simulink model "Tim1PWM_Tim3IC"  (R2018b)
settings: Solver=FixedStepDiscrete  StartTime=0.0  StopTime=10.0  FixedStep=0.5  RelTol=1e-3  EnableMultiTasking=on
libraries: USART_Lib x4, TIMERS_Lib x2, STM32_Config_Lib x1
settings Model: Creator=Gang  LastModifiedBy=fenard1
settings DataIOCC: LimitDataPoints=on  SaveFormat=Array
settings OptimizationCC: DefaultParameterBehavior=Inlined  DefaultUnderspecifiedDataType=single  PassReuseOutputArgsAs=Individual arguments  LifeSpan=1
settings DebuggingCC: UnderspecifiedInitializationDetection=Classic  MergeDetectMultiDrivingBlocksExec=none  SolverPrmCheckMsg=warning  UniqueDataStoreMsg=error  AssertControl=DisableAll  AllowSymbolicDim=off  StrictBusMsg=ErrorOnBusTreatedAsVector  SFUnexpectedBacktrackingDiag=warning  SFNoUnconditionalDefaultTransitionDiag=warning  SFUndirectedBroadcastEventsDiag=error  SFExecutionAtInitializationDiag=none
settings HardwareCC: ProdBitPerPointer=32  ProdBitPerSizeT=32  ProdBitPerPtrDiffT=32  ProdLargestAtomicInteger=Integer  ProdWordSize=32  ProdHWDeviceType=STMicroelectronics->STM32 32-bit Cortex-M
settings ModelReferenceCC: PropagateSignalLabelsOutOfModel=off
settings SFSimCC: SimUseLocalCustomCode=off  CompileTimeRecursionLimit=0  EnableRuntimeRecursion=off  MATLABDynamicMemAlloc=off
settings RTWCC: SystemTargetFile=stm32.tlc  TemplateMakefile=stm32.tmf  Description=stm32 (Embedded Target)  GenerateReport=on  RTWUseLocalCustomCode=off
settings CodeAppCC: IgnoreCustomStorageClasses=off  CustomSymbolStrType=$N$R$M  SimulinkBlockComments=off
settings STFCustomTargetCC: TargetLangStandard=C99 (ISO)  ParMdlRefBuildCompliant=on  IncludeMdlTerminateFcn=off  CombineOutputUpdateFcns=on  ERTCustomFileBanners=on  SupportComplex=off  SupportContinuousTime=off  SupportNonInlinedSFcns=off  RemoveResetFunc=on  ParenthesesLevel=Maximum  CastingMode=Standards  MATLABClassNameForMDSCustomization=Simulink.SoftwareTarget.ERTCustomization  SystemTargetFile=stm32.tlc
settings ERTTargetCC: TargetLangStandard=C99 (ISO)  MultiwordLength=2048  CompOptLevelCompliant=off  ConcurrentExecutionCompliant=off  IncludeMdlTerminateFcn=off  SupportComplex=off  ParenthesesLevel=Maximum  CastingMode=Standards  ModelStepFunctionPrototypeControlCompliant=off  CPPClassGenCompliant=off  UseToolchainInfoCompliant=off  ERTSrcFileBannerTemplate=sourceFileTemplate.cgt  ERTHdrFileBannerTemplate=sourceFileTemplate.cgt  ERTDataSrcFileTemplate=sourceFileTemplate.cgt  ERTDataHdrFileTemplate=sourceFileTemplate.cgt  ERTCustomFileTemplate=customRoutineProcess.tlc  ConvertIfToSwitch=off  SuppressUnreachableDefaultCases=off  EnableSignedLeftShifts=off  EnableSignedRightShifts=off
settings ConfigComp: CovMetricSettings=dw  CovHtmlReporting=on  CovSaveCumulativeToWorkspaceVar=on  CovSaveSingleToWorkspaceVar=on  CovExternalEMLEnable=off  CovSFcnEnable=off

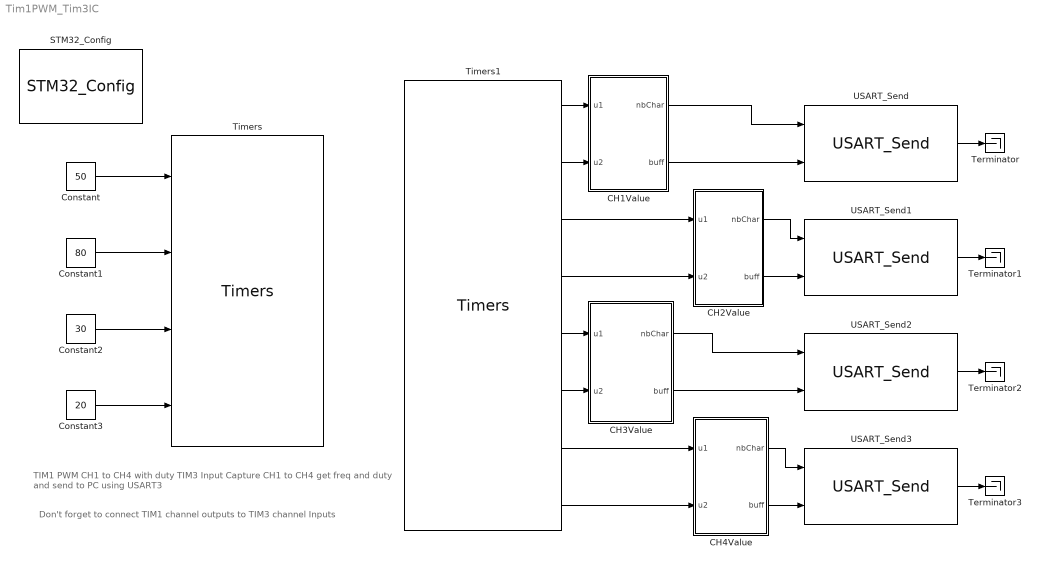
== system Tim1PWM_Tim3IC ==
  note: Don't forget to connect TIM1 channel outputs to TIM3 channel Inputs
  note: TIM1 PWM CH1 to CH4 with duty
      | TIM3 Input Capture CH1 to CH4 get freq and duty and send to PC using USART3
  CH1Value : MATLAB Function  TreatAsAtomicUnit=on
  CH2Value : MATLAB Function  TreatAsAtomicUnit=on
  CH3Value : MATLAB Function  TreatAsAtomicUnit=on
  CH4Value : MATLAB Function  TreatAsAtomicUnit=on
  Constant : Constant  Value=50
  Constant1 : Constant  Value=80
  Constant2 : Constant  Value=30
  Constant3 : Constant  Value=20
  STM32_Config : STM32_Config_Lib/STM32_Config  Priority=0  Project_Path=.\  Config_File=Tim1PWM_Tim3IC.ioc  MCU_Name=STM32F407VGTx
      settings: SourceProductName=Target Support Package - STM32 Adapter
  Terminator{,1..3} (4 alike) : Terminator
  Timers : TIMERS_Lib/Timers  currentTIM=TIM1  TIM_Name=TIM1  sysUsingTimer=on  TIM_APBClock=84000000  TIM_Set_Clk=on  TIM_Prescaler=1  TIM_Clock=42000000.00  Variable_frequency=off  TIM_Set_OutFreq=on  TIM_ARR=2100  Output_frequency=20000.00  Repetition_counter=0  TIM_Mode=Up  TIM_DMA=none  TIM_IRQ=off  TIM_IRQ_ONLY=off  TIM_UP=off  TIM_TRG=off  TIM_COM=off  TIM_BRK=off  NbTIM=2  CH1_enable=on  CH1N_enable=on  CH1_type=Output_PWM  CH1_DMA=off  CH1_int=off  CH1_edge=Rising  CH1_div=1  CH1_variable_duty=on  CH1_set_pulse=off  CH1_output_duty=0.00  CH1_pulse=0  CH2_enable=on  CH2N_enable=on  CH2_type=Output_PWM  CH2_DMA=off  CH2_int=off  CH2_edge=Rising  CH2_div=1  CH2_variable_duty=on  CH2_set_pulse=off  CH2_output_duty=0.00  CH2_pulse=0  CH3_enable=on  CH3N_enable=on  CH3_type=Output_PWM  CH3_DMA=off  CH3_int=off  CH3_edge=Rising  CH3_div=1  CH3_variable_duty=on  CH3_set_pulse=off  CH3_output_duty=0.00  CH3_pulse=0  CH4_enable=on  CH4N_enable=off  CH4_type=Output_PWM  CH4_DMA=off  CH4_int=off  CH4_edge=Rising  CH4_div=1  CH4_variable_duty=on  CH4_set_pulse=off  CH4_output_duty=0.00  CH4_pulse=0
      settings: SourceProductName=Target Support Package - STM32 Adapter
  Timers1 : TIMERS_Lib/Timers  currentTIM=TIM3  TIM_Name=TIM3  sysUsingTimer=on  TIM_APBClock=84000000  TIM_Set_Clk=off  TIM_Prescaler=0  TIM_Clock=84000000.00  Variable_frequency=off  TIM_Set_OutFreq=off  TIM_ARR=1  Output_frequency=84000000.00  Repetition_counter=0  TIM_Mode=Up  TIM_DMA=none  TIM_IRQ=on  TIM_IRQ_ONLY=off  TIM_UP=off  TIM_TRG=off  TIM_COM=off  TIM_BRK=off  NbTIM=2  CH1_enable=on  CH1N_enable=off  CH1_type=Input_Capture  CH1_DMA=off  CH1_int=on  CH1_edge=Rising  CH1_div=1  CH1_variable_duty=on  CH1_set_pulse=off  CH1_output_duty=0.00  CH1_pulse=0  CH2_enable=on  CH2N_enable=off  CH2_type=Input_Capture  CH2_DMA=off  CH2_int=on  CH2_edge=Rising  CH2_div=1  CH2_variable_duty=on  CH2_set_pulse=off  CH2_output_duty=0.00  CH2_pulse=0  CH3_enable=on  CH3N_enable=off  CH3_type=Input_Capture  CH3_DMA=off  CH3_int=on  CH3_edge=Rising  CH3_div=1  CH3_variable_duty=on  CH3_set_pulse=off  CH3_output_duty=0.00  CH3_pulse=0  CH4_enable=on  CH4N_enable=off  CH4_type=Input_Capture  CH4_DMA=off  CH4_int=on  CH4_edge=Rising  CH4_div=1  CH4_variable_duty=on  CH4_set_pulse=off  CH4_output_duty=0.00  CH4_pulse=0
      settings: SourceProductName=Target Support Package - STM32 Adapter
  USART_Send{,1..3} (4 alike) : USART_Lib/USART_Send  USART_name=USART3  Buff_size=512  nbUsart=1  usartMode=Asynchronous  usartDma_Rx=off  usartDma_Tx=off  usartIt=on
      settings: SourceProductName=Target Support Package - STM32 Adapter
  wires:
  Constant/1 -> Timers/1
  Constant1/1 -> Timers/2
  Constant2/1 -> Timers/3
  Constant3/1 -> Timers/4
  CH1Value/1(nbChar) -> USART_Send/1
  CH1Value/2(buff) -> USART_Send/2
  CH2Value/1(nbChar) -> USART_Send1/1
  CH2Value/2(buff) -> USART_Send1/2
  CH3Value/1(nbChar) -> USART_Send2/1
  CH3Value/2(buff) -> USART_Send2/2
  CH4Value/1(nbChar) -> USART_Send3/1
  CH4Value/2(buff) -> USART_Send3/2
  Timers1/1 -> CH1Value/1(u1)
  Timers1/2 -> CH1Value/2(u2)
  Timers1/3 -> CH2Value/1(u1)
  Timers1/4 -> CH2Value/2(u2)
  Timers1/5 -> CH3Value/1(u1)
  Timers1/6 -> CH3Value/2(u2)
  Timers1/7 -> CH4Value/1(u1)
  Timers1/8 -> CH4Value/2(u2)
  USART_Send/1 -> Terminator/1
  USART_Send1/1 -> Terminator1/1
  USART_Send2/1 -> Terminator2/1
  USART_Send3/1 -> Terminator3/1

== matlab function Tim1PWM_Tim3IC/CH2Value ==
  data: u1 input; nbChar output uint16 size=1; buff output uint32 size=1; u2 input
function [nbChar, buff] = convert(u1, u2)
if coder.target('Sfun')
    % Executing in MATLAB, Buff is null
    buff = uint32(0);
    nbChar = uint16(0);
else
    coder.cinclude('stdio.h');
    coder.cinclude('main.h');
    coder.cinclude('getBuffPtr.h');
    % Executing in the generated code.
    ch2Msg = char(zeros(1,30));
    stringSize = uint16(size(ch2Msg,2));
    stringFormat = char(['CH2: %3.3fKHz : %3.3f%%', 13, 10, 0]);
    coder.ceval('snprintf',coder.wref(ch2Msg),stringSize,coder.rref(stringFormat),u1/1000.0,u2);

    buff = coder.ceval('getBuffPtr',coder.rref(ch2Msg));
    nbChar = coder.ceval('strlen',coder.ref(ch2Msg));
end
end

== matlab function Tim1PWM_Tim3IC/CH1Value ==
  data: u1 input; nbChar output uint16 size=1; buff output uint32 size=1; u2 input
function [nbChar, buff] = convert(u1, u2)
if coder.target('Sfun')
    % Executing in MATLAB, Buff is null
    buff = uint32(0);
    nbChar = uint16(0);
else
    coder.cinclude('stdio.h');
    coder.cinclude('main.h');
    coder.cinclude('getBuffPtr.h');
    % Executing in the generated code.
    ch1Msg = char(zeros(1,30));
    stringSize = uint16(size(ch1Msg,2));
    stringFormat = char(['CH1: %3.3fKHz : %3.3f%%', 13, 10, 0]);
    coder.ceval('snprintf',coder.wref(ch1Msg),stringSize,coder.rref(stringFormat),u1/1000.0,u2);

    buff = coder.ceval('getBuffPtr',coder.rref(ch1Msg));
    nbChar = coder.ceval('strlen',coder.ref(ch1Msg));
end
end

== matlab function Tim1PWM_Tim3IC/CH3Value ==
  data: u1 input; nbChar output uint16 size=1; buff output uint32 size=1; u2 input
function [nbChar, buff] = convert(u1, u2)
if coder.target('Sfun')
    % Executing in MATLAB, Buff is null
    buff = uint32(0);
    nbChar = uint16(0);
else
    coder.cinclude('stdio.h');
    coder.cinclude('main.h');
    coder.cinclude('getBuffPtr.h');
    % Executing in the generated code.
    ch3Msg = char(zeros(1,30));
    stringSize = uint16(size(ch3Msg,2));
    stringFormat = char(['CH3: %3.3fKHz : %3.3f%%', 13, 10, 0]);
    coder.ceval('snprintf',coder.wref(ch3Msg),stringSize,coder.rref(stringFormat),u1/1000.0,u2);

    buff = coder.ceval('getBuffPtr',coder.rref(ch3Msg));
    nbChar = coder.ceval('strlen',coder.ref(ch3Msg));
end
end

== matlab function Tim1PWM_Tim3IC/CH4Value ==
  data: u1 input; nbChar output uint16 size=1; buff output uint32 size=1; u2 input
function [nbChar, buff] = convert(u1, u2)
if coder.target('Sfun')
    % Executing in MATLAB, Buff is null
    buff = uint32(0);
    nbChar = uint16(0);
else
    coder.cinclude('stdio.h');
    coder.cinclude('main.h');
    coder.cinclude('getBuffPtr.h');
    % Executing in the generated code.
    ch4Msg = char(zeros(1,30));
    stringSize = uint16(size(ch4Msg,2));
    stringFormat = char(['CH4: %3.3fKHz : %3.3f%%', 13, 10, 0]);
    coder.ceval('snprintf',coder.wref(ch4Msg),stringSize,coder.rref(stringFormat),u1/1000.0,u2);

    buff = coder.ceval('getBuffPtr',coder.rref(ch4Msg));
    nbChar = coder.ceval('strlen',coder.ref(ch4Msg));
end
end
